simulink model "check_modelcompare_drive"  (R2018b)
settings: configuration reference "Physics" (kept outside this file)
libraries: simulink x8
settings Model: DataDictionary=check_modelcompare.sldd  OrderedModelArguments=off  Creator=wischnewski  LastModifiedBy=ga25xiw

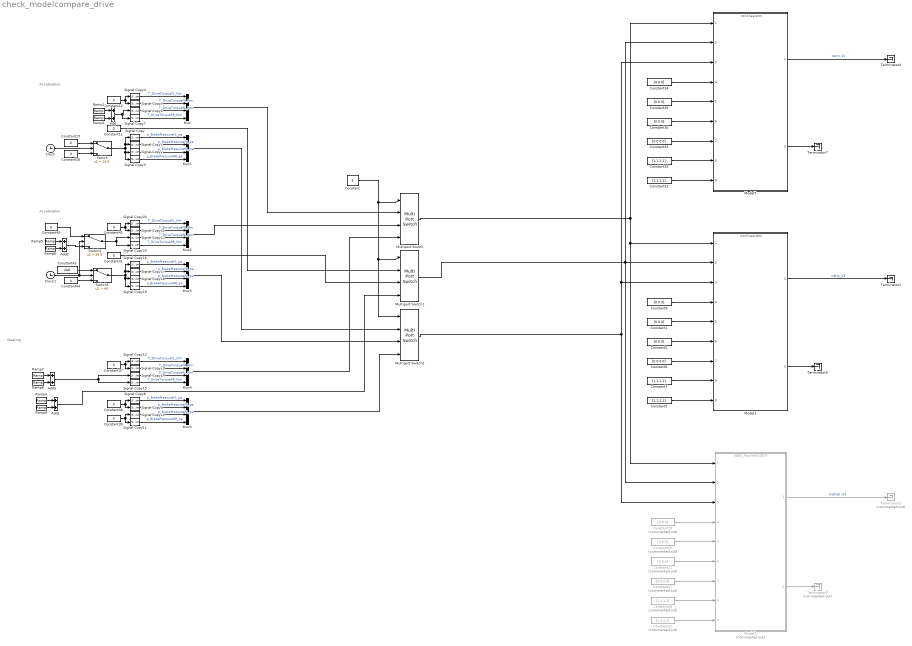
== system check_modelcompare_drive ==
  note: Acceleration
  note: Steering
  note: Acceleration
  Add{,1..3} (4 alike) : Sum
  Clock : Clock
  Clock1 : Clock
  Constant : Constant  Value=3
  Constant{1..2,9,29..30,34} (6 alike) : Constant  Value=[0 0 0]
  Constant{11..12,15..16,37..39,41..42,44..45} (11 alike) : Constant  Value=0
  Constant17 : Constant  Commented=on  Value=[0 0 0 0]
  Constant18 : Constant  Commented=on  Value=[1,1,1,1]
  Constant19 : Constant  Commented=on  Value=[0 0 0]
  Constant20 : Constant  Commented=on  Value=[0 0 0]
  Constant21 : Constant  Commented=on  Value=[0 0 0]
  Constant22 : Constant  Commented=on  Value=[1,1,1,1]
  Constant{5,7,31,33} (4 alike) : Constant  Value=[1,1,1,1]
  Constant32 : Constant  Value=[0 0 0 0]
  Constant43 : Constant  Value=2e6
  Constant6 : Constant  Value=[0 0 0 0]
  Model2 : ModelReference  Commented=on  ModelNameDialog=VDBS_PassVeh14DOF.slx  SimulationMode=Normal  ModelReferenceVersion=1.286
  Model3 : ModelReference  ModelNameDialog=nonlineardtm  ParameterArgumentNames=x0_initialstates  ParameterArgumentValues=[0,0,0,0,0,0]  UsingDefaultArgumentValue=0  SimulationMode=Normal  ModelReferenceVersion=1.737
  Model5 : ModelReference  ModelNameDialog=nonlinearstm  ParameterArgumentNames=x0_positionstates  ParameterArgumentValues=[0,0,0]  UsingDefaultArgumentValue=0  SimulationMode=Normal  ModelReferenceVersion=1.404
  Multiport Switch : MultiPortSwitch
  Multiport Switch1 : MultiPortSwitch
  Multiport Switch2 : MultiPortSwitch
  Mux{,1..5} (6 alike) : Mux
  Ramp1 : simulink/Sources/Ramp  slope=150  start=20  InitialOutput=0
  Ramp2 : simulink/Sources/Ramp  slope=-150  start=30  InitialOutput=0
  Ramp4 : simulink/Sources/Ramp  slope=-0.10  start=30  InitialOutput=0
  Ramp5 : simulink/Sources/Ramp  slope=150  start=20  InitialOutput=0
  Ramp6 : simulink/Sources/Ramp  slope=-150  start=30  InitialOutput=0
  Ramp7 : simulink/Sources/Ramp  slope=100  start=10  InitialOutput=0
  Ramp8 : simulink/Sources/Ramp  slope=-100  start=20  InitialOutput=0
  Ramp9 : simulink/Sources/Ramp  slope=0.10  start=32  InitialOutput=0
  Signal Copy{,1..23} (24 alike) : SignalConversion  OverrideOpt=off
  Switch : Switch  Criteria=u2 > Threshold  Threshold=19.9
  Switch1 : Switch  Criteria=u2 > Threshold  Threshold=40
  Switch2 : Switch  Criteria=u2 > Threshold  Threshold=39.9
  Terminator{1,4,6..7} (4 alike) : Terminator
  Terminator2 : Terminator  Commented=on
  Terminator3 : Terminator  Commented=on
  wires:
  Constant9/1 -> Model3/4
  Constant1/1 -> Model3/5
  Constant2/1 -> Model3/6
  Constant5/1 -> Model3/9
  Constant6/1 -> Model3/7
  Ramp1/1 -> Add/1
  Ramp2/1 -> Add/2
  Constant7/1 -> Model3/8
  Signal Copy2/1 -> Mux1/3  "p_BrakePressureRL_pa"
  Signal Copy/1 -> Mux1/1  "p_BrakePressureFL_pa"
  Signal Copy1/1 -> Mux1/2  "p_BrakePressureFR_pa"
  Multiport Switch2/1 -> Model5/3, Model3/3, Model2/3
  Multiport Switch1/1 -> Model5/2, Model2/2, Model3/2
  Multiport Switch/1 -> Model2/1, Model3/1, Model5/1
  Signal Copy5/1 -> Mux/2  "T_DriveTorqueFR_Nm"
  Signal Copy7/1 -> Mux/4  "T_DriveTorqueRR_Nm"
  Signal Copy4/1 -> Mux/1  "T_DriveTorqueFL_Nm"
  Signal Copy6/1 -> Mux/3  "T_DriveTorqueRL_Nm"
  Signal Copy3/1 -> Mux1/4  "p_BrakePressureRR_pa"
  Constant12/1 -> Signal Copy4/1, Signal Copy5/1
  Switch/1 -> Signal Copy/1, Signal Copy1/1, Signal Copy2/1, Signal Copy3/1
  Model3/1 -> Terminator1/1  "ndtm_V1"
  Constant15/1 -> Switch/1
  Clock/1 -> Switch/2
  Constant16/1 -> Switch/3
  Constant19/1 -> Model2/4
  Constant21/1 -> Model2/6
  Constant18/1 -> Model2/8
  Constant20/1 -> Model2/5
  Constant22/1 -> Model2/9
  Constant17/1 -> Model2/7
  Model2/1 -> Terminator2/1  "matlab std"
  Add/1 -> Signal Copy7/1, Signal Copy6/1
  Constant31/1 -> Model5/9
  Constant34/1 -> Model5/4
  Constant30/1 -> Model5/6
  Constant33/1 -> Model5/8
  Constant29/1 -> Model5/5
  Constant32/1 -> Model5/7
  Model5/1 -> Terminator4/1  "nstm_V2"
  Signal Copy11/1 -> Mux3/4  "p_BrakePressureRR_pa"
  Signal Copy10/1 -> Mux3/3  "p_BrakePressureRL_pa"
  Constant38/1 -> Signal Copy9/1, Signal Copy8/1
  Signal Copy14/1 -> Mux4/3  "T_DriveTorqueRL_Nm"
  Signal Copy12/1 -> Mux4/1  "T_DriveTorqueFL_Nm"
  Constant39/1 -> Signal Copy11/1, Signal Copy10/1
  Signal Copy13/1 -> Mux4/2  "T_DriveTorqueFR_Nm"
  Signal Copy9/1 -> Mux3/2  "p_BrakePressureFR_pa"
  Signal Copy15/1 -> Mux4/4  "T_DriveTorqueRR_Nm"
  Signal Copy8/1 -> Mux3/1  "p_BrakePressureFL_pa"
  Constant37/1 -> Signal Copy12/1, Signal Copy13/1
  Constant/1 -> Multiport Switch2/1, Multiport Switch1/1, Multiport Switch/1
  Mux/1 -> Multiport Switch/2
  Mux4/1 -> Multiport Switch/4
  Constant11/1 -> Multiport Switch1/2
  Add1/1 -> Multiport Switch1/4
  Mux1/1 -> Multiport Switch2/2
  Mux3/1 -> Multiport Switch2/4
  Constant42/1 -> Signal Copy20/1, Signal Copy21/1
  Signal Copy23/1 -> Mux2/4  "T_DriveTorqueRR_Nm"
  Clock1/1 -> Switch1/2, Switch2/2
  Constant43/1 -> Switch1/1
  Signal Copy19/1 -> Mux5/4  "p_BrakePressureRR_pa"
  Signal Copy21/1 -> Mux2/2  "T_DriveTorqueFR_Nm"
  Signal Copy16/1 -> Mux5/1  "p_BrakePressureFL_pa"
  Signal Copy18/1 -> Mux5/3  "p_BrakePressureRL_pa"
  Constant44/1 -> Switch1/3
  Signal Copy22/1 -> Mux2/3  "T_DriveTorqueRL_Nm"
  Signal Copy17/1 -> Mux5/2  "p_BrakePressureFR_pa"
  Signal Copy20/1 -> Mux2/1  "T_DriveTorqueFL_Nm"
  Switch1/1 -> Signal Copy16/1, Signal Copy17/1, Signal Copy18/1, Signal Copy19/1
  Mux5/1 -> Multiport Switch2/3
  Constant41/1 -> Multiport Switch1/3
  Mux2/1 -> Multiport Switch/3
  Ramp5/1 -> Add2/1
  Ramp6/1 -> Add2/2
  Add2/1 -> Switch2/3
  Switch2/1 -> Signal Copy23/1, Signal Copy22/1
  Constant45/1 -> Switch2/1
  Ramp7/1 -> Add3/1
  Ramp8/1 -> Add3/2
  Add3/1 -> Signal Copy14/1, Signal Copy15/1
  Ramp9/1 -> Add1/2
  Ramp4/1 -> Add1/1
  Model2/2 -> Terminator3/1
  Model3/2 -> Terminator6/1
  Model5/2 -> Terminator7/1
